simulink model "Lab2Task2"  (R2016a)
settings: Solver=VariableStepAuto  StartTime=0.0  StopTime=10.0  RelTol=1e-3
settings Model: Creator=Thomas  LastModifiedBy=Thomas

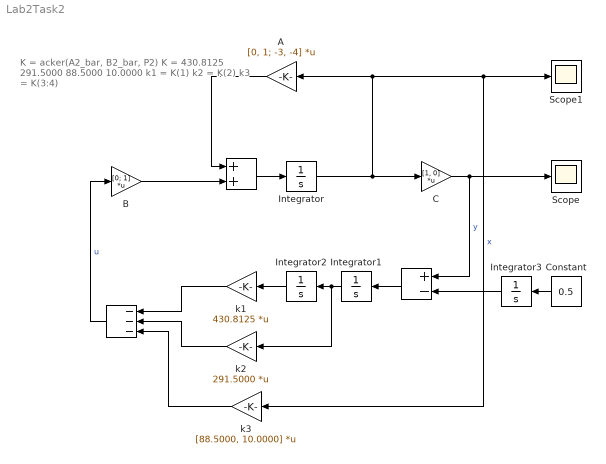
== system Lab2Task2 ==
  note: K = acker(A2_bar, B2_bar, P2)
      | K =  430.8125  291.5000   88.5000   10.0000
      | k1 = K(1)
      | k2 = K(2)
      | k3 = K(3:4)
  " " : Sum  Inputs=+-
  "  " : Sum  Inputs=---
  "   " : Sum
  A : Gain  Gain=[0, 1; -3, -4]  Multiplication=Matrix(K*u)
  B : Gain  Gain=[0; 1]  Multiplication=Matrix(K*u)
  C : Gain  Gain=[1, 0]  Multiplication=Matrix(K*u)
  Constant : Constant  Value=0.5
  Integrator : Integrator  InitialCondition=[0.3;0.4]
  Integrator1 : Integrator
  Integrator2 : Integrator
  Integrator3 : Integrator
  Scope : Scope
  Scope1 : Scope
  k1 : Gain  Gain=430.8125  Multiplication=Matrix(K*u)
  k2 : Gain  Gain=291.5000  Multiplication=Matrix(K*u)
  k3 : Gain  Gain=[88.5000, 10.0000]  Multiplication=Matrix(K*u)
  wires:
  "   "/1 -> Integrator/1
  A/1 -> "   "/1
  B/1 -> "   "/2
  Integrator/1 -> A/1, k3/1, Scope1/1, C/1  "x"
  C/1 -> " "/1, Scope/1  "y"
  k1/1 -> "  "/1
  "  "/1 -> B/1  "u"
  k2/1 -> "  "/2
  Integrator3/1 -> " "/2
  Constant/1 -> Integrator3/1
  k3/1 -> "  "/3
  " "/1 -> Integrator1/1
  Integrator2/1 -> k1/1
  Integrator1/1 -> k2/1, Integrator2/1
